simulink model "full_bridge_invertor_using_mosfet_in_matlab"  (R2018a)
settings: Solver=VariableStepAuto  StartTime=0.0  StopTime=10.0  RelTol=1e-3
libraries: powerlib x8, powerlib_meascontrol x1
settings Model: Creator=pursh  LastModifiedBy=pursh

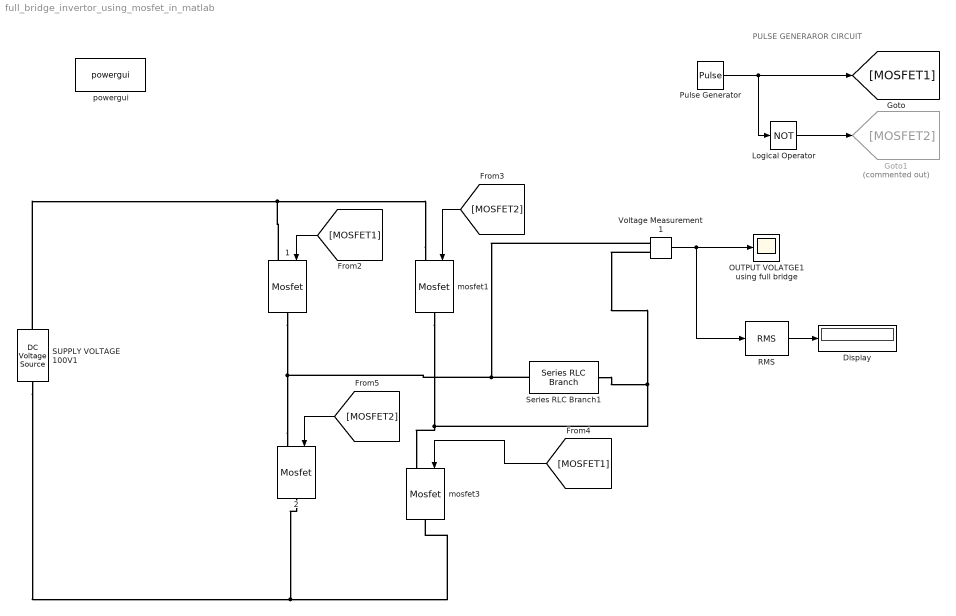
== system full_bridge_invertor_using_mosfet_in_matlab ==
  note: PULSE GENERAROR CIRCUIT
  " 1" : powerlib/Power Electronics/Mosfet  Ron=0.1  Lon=0  Rd=0.01  Vfd=0  IC=0  Rs=1e5  Cs=inf  Measurements=off
  " 2" : powerlib/Power Electronics/Mosfet  Ron=0.1  Lon=0  Rd=0.01  Vfd=0  IC=0  Rs=1e5  Cs=inf  Measurements=off
  Display : Display
  Goto1 : Goto  Commented=on  GotoTag=MOSFET2
  Logical Operator : Logic  Operator=NOT  AllPortsSameDT=off  OutDataTypeStr=boolean
  "OUTPUT VOLATGE1 using full bridge " : Scope
  Pulse Generator : DiscretePulseGenerator  PulseType=Time based  Period=2e-5  PulseWidth=50
  RMS : powerlib_meascontrol/Measurements/RMS  TrueRMS=on  Freq=60  RMSInit=120  Ts=0
  SUPPLY VOLTAGE 100V1 : powerlib/Electrical Sources/DC Voltage Source  Amplitude=100  Measurements=None
  Series RLC Branch1 : powerlib/Elements/Series RLC Branch  LConnTagsString=__new0  RConnTagsString=__new0  BranchType=R  Resistance=50  Inductance=1e-3  SetiL0=off  InitialCurrent=0  Capacitance=1e-6  Setx0=off  InitialVoltage=0  Measurements=None
  Voltage Measurement1 : powerlib/Measurements/Voltage Measurement  PhasorSimulation=off  OutputType=Complex  PSBequivalent=0
  mosfet1 : powerlib/Power Electronics/Mosfet  Ron=0.1  Lon=0  Rd=0.01  Vfd=0  IC=0  Rs=1e5  Cs=inf  Measurements=off
  mosfet3 : powerlib/Power Electronics/Mosfet  Ron=0.1  Lon=0  Rd=0.01  Vfd=0  IC=0  Rs=1e5  Cs=inf  Measurements=off
  powergui : powerlib/powergui  Priority=1  SimulationMode=Continuous  SampleTime=50e-6  frequency=60  Iterations=50  frequencyindice=0  Pbase=100e6  ErrMax=1e-4  UnitsV=kV  UnitsW=MW  buscounter=0  FunctionMessages=off  echomessages=off  EnableUseOfTLC=off  CurrentSourceSwitches=off  DisableSnubberDevices=off  DisableRonSwitches=off  DisableVfSwitches=off  DisplayEquations=off  SolverType=Tustin/Backward Euler (TBE)  Interpol=off  ExternalGateDelay=off  methode=off  Ts=100  x0status=blocks  SPID=on  SwTol=0  HookPort=off  RestoreLinks=warning  ResistiveCurrentMeasurement=off  Frange=[0:2:500]  Ylog=off  Xlog=on  ShowGrid=off  save=off  variable=ZData  structure=0  ZoomFFT=off  StartTime=0.0  cycles=1  DisplayStyle=1  fundamental=60  FreqAxis=off  MaxFrequency=1000  frequencyindicesteady=1  RmsSteady=1  display=off
  wires:
  RMS/1 -> Display/1
  [MOSFET2] -> mosfet1/1
  [MOSFET2] -> " 2"/1
  [MOSFET1] -> mosfet3/1
  Voltage Measurement1/1 -> RMS/1, "OUTPUT VOLATGE1 using full bridge "/1
  [MOSFET1] -> " 1"/1
  Pulse Generator/1 -> Logical Operator/1, [MOSFET1]
  Logical Operator/1 -> Goto1/1
  connections:
  " 2"/LConn1 -- " 1"/RConn1 -- Voltage Measurement1/LConn1 -- Series RLC Branch1/LConn1
  mosfet3/RConn1 -- SUPPLY VOLTAGE 100V1/LConn1 -- " 2"/RConn1
  Voltage Measurement1/LConn2 -- Series RLC Branch1/RConn1 -- mosfet1/RConn1 -- mosfet3/LConn1
  mosfet1/LConn1 -- SUPPLY VOLTAGE 100V1/RConn1 -- " 1"/LConn1
